simulink model "FSK"  (R2023b)
settings: Solver=VariableStepAuto  StartTime=0.0  StopTime=30  RelTol=1e-3
settings Model: Creator=HP  LastModifiedBy=HP

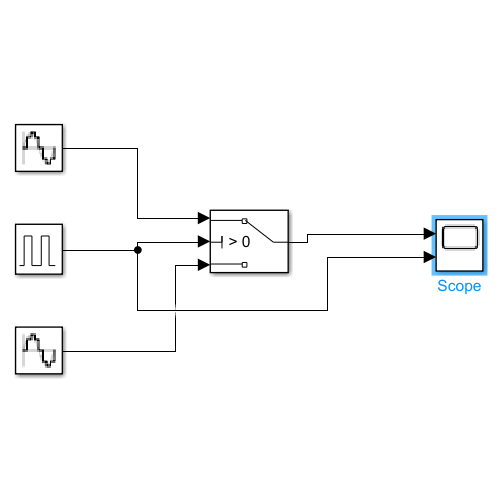
[thumbnail: Simulink's stored preview of the top-level diagram]
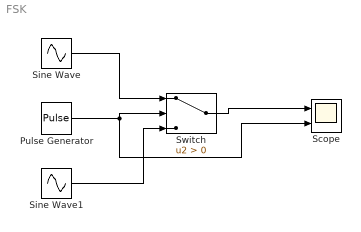
== system FSK ==
  Pulse Generator : DiscretePulseGenerator  PulseType=Time based  Period=5  PulseWidth=5
  Scope : Scope  NumInputPorts=2
  Sine Wave : Sin  Frequency=80  SampleTime=0.01
  Sine Wave1 : Sin  Frequency=10  SampleTime=0.01
  Switch : Switch  Criteria=u2 > Threshold  SaturateOnIntegerOverflow=off  InputSameDT=off
  wires:
  Switch/1 -> Scope/1
  Pulse Generator/1 -> Scope/2, Switch/2
  Sine Wave1/1 -> Switch/3
  Sine Wave/1 -> Switch/1
